simulink model "part2"  (R2019b)
settings: Solver=FixedStepAuto  StartTime=0.0  StopTime=1000  FixedStep=0.1  RelTol=1e-3
values from neighbouring files (symbols this model uses):
  A_w = [zeros(3) eye(3) ... (first row only)    [initObs.m]
  B_pseudo = inv(W)*B_u'*inv(B_u*inv(W)*B_u' + epsilon.*eye(3))    [init_thrustAloc.m]
  C_w = [zeros(3) eye(3)]    [initObs.m]
  constant_dp = 0    [pick_sp.m]
  corner_test = 0    [pick_sp.m]
  corners = [0,0,0;50,0,0;50,-50,0;50,-50,-pi/4;0,-50,-pi/4;0,0,0]    [pick_sp.m]
  curr_mean_dir = curr_mean_dir + 10    (= 10)    [capabilitytest.m]    (also in pick_sp.m = 270)
  curr_mean_vel = 0.2    [pick_sp.m]
  D = diag([2.6486e+05,8.8164e+05,3.3774e+08])    [init.m]    (also in initObs.m = [2.648*10^5 0 0)
  Delta_stack = zeros(15,3,360)    [init_kalman.m]
  Gamma_stack = zeros(15,6,360)    [init_kalman.m]
  H = [Cw, eye(3),zeros(3,6)]    [init_kalman.m]
  K1 = [-2*(zeta_ni_nop - zeta_i_nop)*(omega_ci_nop/omega_p)*eye(3) ... (first row only)    [initObs.m]
  K2 = diag([omega_ci_nop omega_ci_nop omega_ci_nop])    [initObs.m]
  K3 = 0.1*K4    [initObs.m]
  K4 = diag([0.1 0.1 0.01])    [initObs.m]
  Kd = [1e+07,1e+07,2.01e+08]    [tune.m]
  Ki = [2e+02,2e+02,1e+02]    [tune.m]
  Kp = [1e+05,5e+05,1e+07]    [tune.m]
  M = [6.8177e+06,0,0;0,7.8784e+06,-2.5955e+06;0,-2.5955e+06,3.57e+09]    [init.m]    (also in initObs.m = [ 6.8177*10^6 0 0)
  observer_on = 1    [pick_sp.m]
  Phi_stack = zeros(15,15,360)    [init_kalman.m]
  Q = diag([Q1 Q2])    [init_kalman.m]
  R_KF = diag([0 0 0])    [init_kalman.m]
  ref_model_on = 1    [pick_sp.m]
  setpoint = [0,0,0]    [pick_sp.m]
  T_b = diag([1000 1000 1000])    [initObs.m]
  thrusters =     [thrusters_sup.mat]
  use_kalman = 1    [pick_sp.m]
  vessel =     [thrusters_sup.mat]
  w_n = [0.08,0.04,0.03]    [tune.m]
  wave_mean_dir = wave_mean_dir + (10*pi/180)    (= 0.174532925199)    [capabilitytest.m]    (also in pick_sp.m = 225)
  wave_peak_T = 13    [pick_sp.m]
  wind_mean_dir = wind_mean_dir + (10*pi/180)    (= 0.174532925199)    [capabilitytest.m]    (also in pick_sp.m = 180)
  wind_mean_vel = 15    [pick_sp.m]
  zeta = 1    [tune.m]
undefined symbols (not defined in the file or in its folder): Hoerner, magnitude
libraries: marine_gnc x13, simulink x4, cstblocks x4, marine_hydro x2
(part 2 of 2)

== matlab function part2/Wind/Convert angle to index in wind_coeff ==
  data: ang input; index output
function index = angle2index(ang)

%ang is the angle difference between the ship and the wind direction
%ang is somewhere in [-pi,pi] and we want an index between 1 & 37
%This index will be used to look up in the wind coefficient matrix

%Convert from [-pi,pi] to [0,2pi]
if (ang >= -pi && ang < 0)
    ang = ang + 2*pi;
end

%Convert to degrees since table data is in degrees
ang = ang*180/pi;

%Round to nearest 10 and add 1 since Matlab indexes from 1 for some reason
index = mod(round(0.1*ang) + 1,37);

== matlab function part2/Reference Model/Setpoint /Corner_test ==
  data: nu input; eta input; corners input; setpoint output; new_setpoint output; setpoint_index input; setpoint_index output
function [setpoint, new_setpoint, setpoint_index] = fcn(nu, eta, corners, setpoint_index)

setpoint=corners(setpoint_index,:);

eta_tol = [0.5,0.5,pi/180];
nu_tol = [0.05,0.05,0.01];

err = [abs(setpoint-eta');abs(nu')];
test = err > [eta_tol;nu_tol];
new_setpoint = 0;
if (sum(sum(test)) == 0)
    setpoint_index = mod(setpoint_index,6)+1;
    % NB: The corner test will loop once finished.
    new_setpoint = 1;
end

== matlab function part2/Observer/Kalman Filter /Extended Kalman Filter/Discrete Kalman Filter ==
  data: P_in input; x_in input; Phi input; Delta input; Gamma input; Q input; R input; H input; u input; P_hat output; y input; x_hat output
%%%%%%%%%%%%%%%%%%%%%%%%%%%%%%%%%%%%%%%%%%%%%%%%%%%%%%%%%%%%%%%%%%%%%%%%%%%
% EKF()                                                                   %
%                                                                         %              
% Implementation of the Extended Kalman algorithm for part2.slx           %
%                                                                         %
% Created:      15.10.2020	                                              %
%                                                                         %
%%%%%%%%%%%%%%%%%%%%%%%%%%%%%%%%%%%%%%%%%%%%%%%%%%%%%%%%%%%%%%%%%%%%%%%%%%%

function [P_hat, x_hat] = EKF(P_in, x_in, Phi, Delta, Gamma, Q, R, H, u, y)

% Predictor
x_bar = Phi*x_in + Delta*u;
P_bar = Phi*P_in*Phi' + Gamma*Q*Gamma';

% Kalman Gain
K = (P_bar*H')*inv(H*P_bar*H' + R);

% Corrector 
x_hat = x_bar + K*(y - H*x_bar);
P_hat = (eye(size(P_bar)) - K*H)*P_bar*(eye(size(P_bar))-K*H)' + K*R*K';

end

== matlab function part2/Thruster Dynamics/MATLAB Function ==
  data: alpha_actual input; thrust_actual input; actual_tau output; PosX input; PosY input
function actual_tau   = fcn(alpha_actual,thrust_actual,PosX,PosY)

    Alpha_surge =[cos(alpha_actual(1)) cos(alpha_actual(2)) cos(alpha_actual(3)) cos(alpha_actual(4)) cos(alpha_actual(5))];  
    Alpha_sway = [sin(alpha_actual(1)) sin(alpha_actual(2)) sin(alpha_actual(3)) sin(alpha_actual(4)) sin(alpha_actual(5))];
    Alpha_yaw = [sin(alpha_actual(1))*PosX(1)-cos(alpha_actual(1))*PosY(1) sin(alpha_actual(2))*PosX(2)-cos(alpha_actual(2))*PosY(2) ...
                 sin(alpha_actual(3))*PosX(3)-cos(alpha_actual(3))*PosY(3) sin(alpha_actual(4))*PosX(4)-cos(alpha_actual(4))*PosY(4) ...
                 sin(alpha_actual(5))*PosX(5)-cos(alpha_actual(5))*PosY(5)];

    actual_tau = [Alpha_surge; Alpha_sway; Alpha_yaw]*thrust_actual;
end

== matlab function part2/Thrust Allocation/QP-algorithm ==
  data: tau_d input; u_in input; u output; alpha output; alpha_in input
function [u, alpha]= Thrust_allocation(tau_d, u_in, alpha_in)
    B = [0, cos(alpha_in(2)), cos(alpha_in(3)), cos(alpha_in(4)), cos(alpha_in(5));
         1, sin(alpha_in(2)), sin(alpha_in(3)), sin(alpha_in(4)), sin(alpha_in(5));
         39.3, 35.3*sin(alpha_in(2)),  31.3*sin(alpha_in(3)), -28.5*sin(alpha_in(4))-5*cos(alpha_in(4)), -28.5*sin(alpha_in(5))+5*cos(alpha_in(5))];
    
    s = [1; 1; 1; 1; 1];
   
    Aeq = [B, -eye(5)]*[u_in; s];
    Aie = [-eye(5), 0; eye(5), 0]*[u_in; s];
    tau_iq = 
    H = 2*diag([1, 10, 10, 10, 10, 100, 100, 100, 100, 100]);
    lb = zeros(1,10)';
    ub = [125, 150, 150, 320, 320, 15.625, 18.75, 18.75, 32, 32]';
    
    u = quadprog(H, 0, B, tau_d, Aeq, tau_d, lb, ub);
    
    q
    
    %Thruster angle

end

== matlab function part2/Thrust Allocation/second try/Shortest rotational path ==
  data: angle_old input; next_angle input; optimal_angle output
function optimal_angle = shortestRoute(angle_old,next_angle)
    % Remainder of difference between desired and reference in 0,2pi. NB:
    % read documentation on mod() to understand what happens with negative
    % first arguments.
    angle_temp = mod((next_angle - angle_old), 2*pi);
    
    % Add 2pi for positive angle, and find the remainder in [0,2pi]
    shortest = mod(angle_temp + 2*pi, 2*pi);
    
    % Map to (-pi,pi] for shortest rotation.
    if (shortest > pi)
        shortest = shortest - 2*pi;
    end   
    
    optimal_angle = angle_old + shortest;
    
    %We also want to apply some nice constraints to the angle:
%     rot_limits = [2 2 2 2].*pi/30; % Rotation limits for azimuths [rad/s]
%     for i = 1:4
%         d_alpha = maybe_angle(i) - angle_old(i);
%         if d_alpha > rot_limits(i)
%             optimal_angle(i) = angle_old(i) + rot_limits(i);
%         elseif d_alpha < -rot_limits(i)
%             optimal_angle(i) = angle_old(i) - rot_limits(i);
%         else 
%             optimal_angle = maybe_angle
%         end
%     end
end

== matlab function part2/Thrust Allocation/second try/Woho ==
  data: u_i input; u output; u_past input
function u = fcn(u_i, u_past)
    u= zeros(1,5)';
    
    u(1) = u_i(1);
    u(2) = sqrt(u_i(2)^2+u_i(3)^2);
    u(3) = sqrt(u_i(4)^2+u_i(5)^2);
    u(4) = sqrt(u_i(6)^2+u_i(7)^2);
    u(5) = sqrt(u_i(8)^2+u_i(9)^2);
    
    ts = 0.1 %timestep
    max_thrust = [125000 150000 150000 320000 320000]; % [N]
    thrust_speed = [8 8 8 10 10]; % From 0 - 100% RPM [s]
    thrust_rate  = max_thrust ./ thrust_speed; % [N/s]
    delta_thrust = ts.*thrust_rate; % [N/timestep]
    
    for i = 1:5
        % Check to see if change in thrust has been violating limitations
        du = u(i) - u_past(i); 
        if du > delta_thrust(i)
            u(i) = u_past(i) + delta_thrust(i);
        elseif du < -delta_thrust(i)
            u(i) = u_past(i) - delta_thrust(i);
        end
        
        % Bound magnitude of thrust
        if u(i) > max_thrust(i)
            u(i) = max_thrust(i);
        elseif u(i) < -max_thrust(i)
            u(i) = -max_thrust(i);
        end
    end
end

== matlab function part2/Thrust Allocation/second try/Angle conversion/Rotation filtering (not working)/Projection  ==
  data: u input; y output; Tfs input
function y = fcn(u, Tfs)
y = (dot(u,Tfs)/ (norm(Tfs)^2)).*Tfs;
if(norm(Tfs) == 0) y = zeros(1,9)';end
end

== matlab function part2/Thrust Allocation/second try/Angle conversion/atan  ==
  data: Tfs input; alpha output
function alpha = fcn(Tfs)
    alpha = [pi/2 0 0 0 0]';
    alpha(2) = atan2(Tfs(2),Tfs(3));
    alpha(3) = atan2(Tfs(4),Tfs(5));
    alpha(4) = atan2(Tfs(6),Tfs(7));
    alpha(5) = atan2(Tfs(8),Tfs(9));
    
    % Eliminate singularities 
%     check = isnan(alpha);
%     for i = 2:length(check)
%         if check(i)
%             alpha(i) = pi;
%         end
%     end    
end

== matlab function part2/Thrust Allocation/MATLAB Function ==
  data: u_ext output; tau_c input
function u_ext  = extended_thrust(tau_c)
% Initialize extended thrust vector

    % Positional value for the thrusters, in meters
    lx = [39.3  35.3    31.3    -28.5   -28.5];
    ly = [0     0       0       5       -5];
    
    % Create thruster configuration matrix for extended thrust method
    t1   = [0 1 lx(1)]';  % Bow tunnel thruster 1 sway and yaw effect
    t2_x = [1 0 ly(2)]';  % Bow azimuth x-component 
    t2_y = [0 1 lx(2)]';  % Bow azimuth y-component
    t3_x = [1 0 ly(3)]';  % Bow azimuth x-component 
    t3_y = [0 1 lx(3)]';  % Bow azimuth y-component
    t4_x = [1 0 ly(4)]';  % Stern azimuth portside x-component 
    t4_y = [0 1 lx(4)]';  % Stern azimuth portside y-component 
    t5_x = [1 0 ly(5)]';  % Stern azimuth starboard x-component 
    t5_y = [0 1 lx(5)]';  % Stern azimuth starboard y-component
    
    T_ext = [t1 t2_x t2_y t3_x t3_y t4_x t4_y t5_x t5_y];
    
    W = diag([1,10,10,10,10,10,10,10,10]); % Cost matrix
    
    % Find pseudo inverse
    sym = T_ext * W^(-1) * T_ext';
    I = eye(size(sym));
    epsilon = 0.1;
    C = W^(-1) * T_ext' * (sym + epsilon.*I)^(-1);
    
    % Get the extended thrust vector
    u_ext = C * tau_c;
end

== matlab function part2/Thrust Allocation/MATLAB Function1 ==
  data: u_prev input; u output; u_ext input; alpha output; alpha_prev input
function [u,alpha] = gang(u_prev, u_ext, alpha_prev)

    Ts              = 0.1;
    max_thrust      = [125000 150000 150000 320000 320000]; % [N]
    thrust_speed    = [8 8 8 10 10]; % From 0 - 100% RPM [s]
    thrust_rate     = max_thrust ./ thrust_speed; % [N/s]
    delta_thrust    = Ts.*thrust_rate; % [N/timestep]
    rot_limits      = [0 2 2 2 2].*pi/30; % Rotation limits for azimuths [rad/s]

% Collect the representation of the real thrust
    u = zeros(5,1);
    u(1) = u_ext(1);
    u(2) = sqrt(u_ext(2)^2 + u_ext(3)^2);
    u(3) = sqrt(u_ext(4)^2 + u_ext(5)^2);
    u(4) = sqrt(u_ext(6)^2 + u_ext(7)^2);
    u(5) = sqrt(u_ext(8)^2 + u_ext(9)^2);

% Calculate the resulting azimuth angles
    alpha = ones(5,1).*pi/2; % Initialize according to tunnel thrusters
    alpha2des = atan2(u_ext(3),u_ext(2));
    alpha3des = atan2(u_ext(5),u_ext(4)); % atan2 naturally maps in -pi,pi,
    alpha4des = atan2(u_ext(7),u_ext(6)); % and fins angle between the y and x
    alpha5des = atan2(u_ext(9),u_ext(8)); % component of the azimuths thrust
    
    % Determine angle based on shortest path between previous angle and desired
    % angle, since the input to the thrusters just follows the number line.  
    alpha(2) = alpha_prev(2) + shortestRot(alpha_prev(2),alpha2des);
    alpha(3) = alpha_prev(3) + shortestRot(alpha_prev(3),alpha3des);
    alpha(4) = alpha_prev(4) + shortestRot(alpha_prev(4),alpha4des);
    alpha(5) = alpha_prev(5) + shortestRot(alpha_prev(5),alpha5des);
      
 %   Check to see if it is better to rotate oppositely, and swich signs
    for i = [2,3,4,5]
        d_alpha = alpha(i) - alpha_prev(i); % angular difference
        
        if d_alpha > pi/2
            alpha(i) = alpha_prev(i) - (pi-(alpha(i)-alpha_prev(i)));
            u(i) = -u(i);
        elseif d_alpha < -pi/2
            alpha(i) = alpha_prev(i) + (pi + (alpha(i)-alpha_prev(i)));
            u(i) = -u(i);
        end
    end

    % Add constraints - performing constrained thrust allocation
    for i = 1:5
        % Check to see if change in thrust has been violating limitations
        du = u(i) - u_prev(i); 
        if du > delta_thrust(i)
            u(i) = u_prev(i) + delta_thrust(i);
        elseif du < -delta_thrust(i)
            u(i) = u_prev(i) - delta_thrust(i);
        end
        
        % Bound magnitude of thrust
        if u(i) > max_thrust(i)
            u(i) = max_thrust(i);
        elseif u(i) < -max_thrust(i)
            u(i) = -max_thrust(i);
        end
    end
    
    % Check rotational constraints
    for i = 2:5
        d_alpha = alpha(i) - alpha_prev(i);
        if d_alpha > rot_limits(i)
            alpha(i) = alpha_prev(i) + rot_limits(i);
        elseif d_alpha < -rot_limits(i)
            alpha(i) = alpha_prev(i) - rot_limits(i);
        end
    end  
end

function out_angle = shortestRot(angle,angle_desired)
    % Remainder of difference between desired and reference in 0,2pi. NB:
    % read documentation on mod() to understand what happens with negative
    % first arguments.
    angle_temp = mod((angle_desired - angle), 2*pi);
    
    % Add 2pi for positive angle, and find the remainder in [0,2pi]
    out_angle = mod(angle_temp + 2*pi, 2*pi);
    
    % Map to (-pi,pi] for shortest rotation.
    if (out_angle > pi)
        out_angle = out_angle - 2*pi;
    end    
end

== matlab function part2/Thrust Allocation/Slowly varying angles/Projection  ==
  data: u input; y output; Tfs input
function y = fcn(u, Tfs)
y = (dot(u,Tfs)/ (norm(Tfs)^2)).*Tfs;
if(norm(Tfs) == 0) y = zeros(1,9)';end
end

== matlab function part2/Observer/Kalman Filter /Extended Kalman Filter/EKF - Linearized parameters ==
  data: x_hat input; Phi output; Delta output; Gamma output; Phi_stack input; Delta_stack input; Gamma_stack input
function [Phi,Delta,Gamma] = fcn(x_hat,Phi_stack,Delta_stack,Gamma_stack)

% Use previous heading to determine rotation matrix for linearization
last_yaw = x_hat(3);
ind = round(last_yaw*pi/180);
if (ind<0) ind = ind+360;end

% Collect the linearized KF parameters (generated by init_kalman.m)
Phi   = Phi_stack(:,:,ind+1);
Delta = Delta_stack(:,:,ind+1);
Gamma = Gamma_stack(:,:,ind+1);

end
